simulink model "SmallFixedWingUAVupperHIL"  (R2022b)
settings: Solver=FixedStepDiscrete  StartTime=0.0  StopTime=inf  FixedStep=1/300  RelTol=1e-3
model workspace: external: MAT-File E:\RFLY\small-fixed-wing-book\fixedwing-book-rfly\ch8\code\e7-4\hitl\desire.mat (data not in the file)
values from neighbouring files (symbols this model uses):
  ctrlpoints = [xd'-xd(1);yd'-yd(1)]    [bspline.m]
  env = struct    [InitDatactrl.m]
  knots = [t1, t2, t3]    [bspline.m]
  pp = 3    [bspline.m]
  uav = struct    [InitDatactrl.m]
undefined symbols (not defined in the file or in its folder): DiscIntNeverNeededParam, RGBLED_COLOR_ENUM, RGBLED_MODE_ENUM
libraries: simulink x10, pixhawk_slib_sensors_actuators x6, pixhawk_slib_uORB_RW x5
(part 1 of 2)
settings Model: Creator=Steve  LastModifiedBy=DELL
settings SolverCC: AlgebraicLoopSolver=TrustRegion  AutoInsertRateTranBlk=on
settings DataIOCC: LimitDataPoints=on  SaveFormat=Array  ReturnWorkspaceOutputs=off
settings OptimizationCC: DefaultParameterBehavior=Inlined  ZeroExternalMemoryAtStartup=off  ZeroInternalMemoryAtStartup=off  LifeSpan=1  MaxStackSize=64  EfficientTunableParamExpr=on
settings DebuggingCC: SolverPrmCheckMsg=warning  UnconnectedInputMsg=warning  UnconnectedOutputMsg=warning  UnconnectedLineMsg=warning  AllowSymbolicDim=off  SFUnexpectedBacktrackingDiag=warning  SFNoUnconditionalDefaultTransitionDiag=warning  SFExecutionAtInitializationDiag=none  SFMachineParentedDataDiag=warning  ArithmeticOperatorsInVariantConditions=warning
settings HardwareCC: ProdBitPerPointer=32  ProdBitPerSizeT=32  ProdBitPerPtrDiffT=32  ProdLargestAtomicInteger=Long  ProdLargestAtomicFloat=Double  ProdWordSize=32  ProdHWDeviceType=ARM Compatible->ARM Cortex
settings ModelReferenceCC: EnableRefExpFcnMdlSchedulingChecks=on  PropagateSignalLabelsOutOfModel=off
settings SFSimCC: SimUseLocalCustomCode=off  MATLABDynamicMemAllocThreshold=0  CustomCodeUndefinedFunction=UseInterfaceOnly
settings RTWCC: Description=Embedded Coder  SystemTargetFile=ert.tlc  HardwareBoard=Pixhawk PX4  TemplateMakefile=ert_default_tmf  GenerateReport=on  RTWUseLocalCustomCode=off  Toolchain=Pixhawk Toolchain  BuildConfiguration=Faster Runs  IncludeHyperlinkInReport=on  LaunchReport=on  GenerateTraceReport=on  GenerateTraceReportSl=on  GenerateTraceReportSf=on  GenerateTraceReportEml=on  GenerateCodeMetricsReport=on  DLArmComputeVersion=19.05
settings CodeAppCC: IgnoreCustomStorageClasses=off  StateflowObjectComments=on
settings ERTTargetCC: TargetLangStandard=C99 (ISO)  CodeReplacementLibrary=GCC ARM Cortex-A9  MultiwordLength=2048  SupportContinuousTime=on  SupportVariableSizeSignals=on  ExtModeTransport=1  ExtModeMexFile=ext_serial_win32_comm  ExtModeMexArgs=/dev/serial  RootIOFormat=Structure reference  ERTCustomFileTemplate=PX4_codertarget_file_process.tlc  ConvertIfToSwitch=off  SuppressUnreachableDefaultCases=off
settings ConfigComp: CovMetricSettings=dw  CovSaveCumulativeToWorkspaceVar=on  CovSaveSingleToWorkspaceVar=on  CovExternalEMLEnable=off  CovSFcnEnable=off

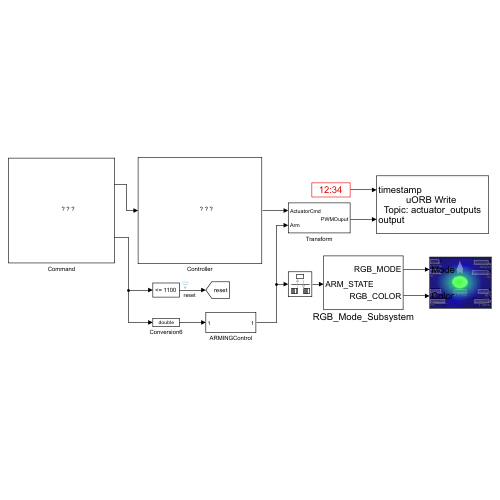
[thumbnail: Simulink's stored preview of the top-level diagram]
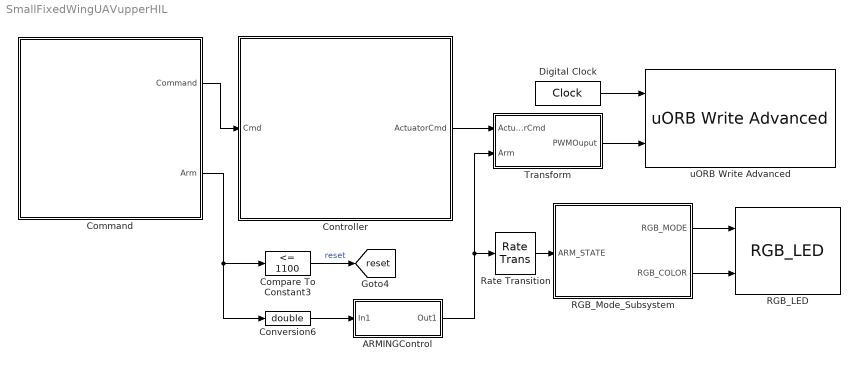
== system SmallFixedWingUAVupperHIL ==
  ARMINGControl : Subsystem
  Command : Subsystem
      mask Display: image('D:\GwhBuaa207\Project\2022-2023FW\fixedwing-book-rfly\chr\code\e0\hil\control\icon\ledi.jpg'); % 使用工具条上的 "编辑图像" 进行更改。
  Compare To Constant3 : simulink/Logic and Bit Operations/Compare To Constant  relop=<=  const=1100  OutDataTypeStr=boolean
  Controller : Subsystem
      mask Display: image('D:\GwhBuaa207\Project\2022-2023FW\fixedwing-book-rfly\chr\code\e0\hil\control\icon\Cube-Orange.jpg'); % 使用工具条上的 "编辑图像" 进行更改。
  Conversion6 : DataTypeConversion  OutDataTypeStr=double  SaturateOnIntegerOverflow=off  RndMeth=Floor
  Digital Clock : DigitalClock  SampleTime=-1
  RGB_LED : pixhawk_slib_sensors_actuators/RGB_LED
      settings: SourceProductName=Pixhawk Target Blocks
  RGB_Mode_Subsystem : Subsystem
  Rate Transition : RateTransition  OutPortSampleTime=1
  Transform : Subsystem
  uORB Write Advanced : pixhawk_slib_uORB_RW/uORB Write Advanced  Ts=0  uORB_AdvtQueue=on  uORB_FieldEnabledArr="0  0  0  1  0  0  0  0  0  0  0"  uORB_Topic_str=0  uORB_Struct_DT="[1  1  1  1  1]"  BlockInputCount=5  uORB_StructParams="[\"voltage_v\",\"voltage_filtered_v\",\"current_a\",\"current_filtered_a\",\"remaining\"]"  uORB_PortSizes="[1  1  1  1]"  MsgSizeOf=0  MW_update=true
      settings: SourceProductName=Pixhawk Target Blocks
  tag scope: reset=global
  wires:
  Digital Clock/1 -> uORB Write Advanced/1
  RGB_Mode_Subsystem/1(RGB_MODE) -> RGB_LED/1
  Rate Transition/1 -> RGB_Mode_Subsystem/1(ARM_STATE)
  ARMINGControl/1(Out1) -> Transform/2(Arm), Rate Transition/1
  RGB_Mode_Subsystem/2(RGB_COLOR) -> RGB_LED/2
  Conversion6/1 -> ARMINGControl/1(In1)
  Compare To Constant3/1 -> [reset]  "reset"
  Transform/1(PWMOuput) -> uORB Write Advanced/2
  Controller/1(ActuatorCmd) -> Transform/1(ActuatorCmd)
  Command/2(Arm) -> Conversion6/1, Compare To Constant3/1
  Command/1(Command) -> Controller/1(Cmd)

== system SmallFixedWingUAVupperHIL/ARMINGControl ==
  In1 : Inport
  Compare To Constant3 : simulink/Logic and Bit Operations/Compare To Constant  relop=>=  const=uint16(1500)  OutDataTypeStr=boolean
  Out1 : Outport  VectorParamsAs1DForOutWhenUnconnected=off
  wires:
  Compare To Constant3/1 -> Out1/1
  In1/1 -> Compare To Constant3/1

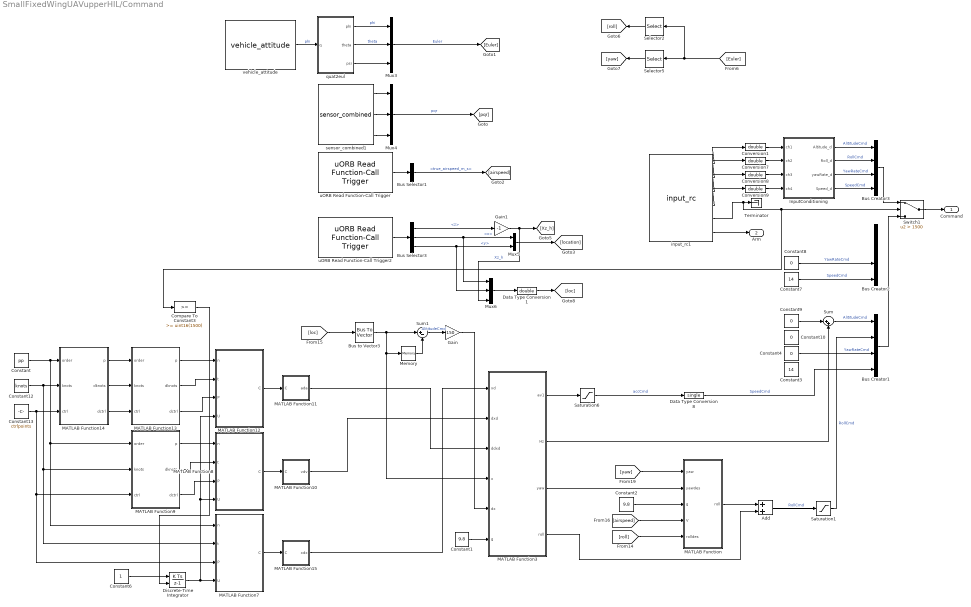
== system SmallFixedWingUAVupperHIL/Command ==
  Add : Sum
  Bus Creator1 : BusCreator  Inputs=4
  Bus Creator2 : BusCreator  Inputs=4
  Bus Creator3 : BusCreator  Inputs=4
  Bus Selector1 : BusSelector  OutputSignals=true_airspeed_m_s
  Bus Selector3 : BusSelector  OutputSignals=z,x,y
  Bus to Vector3 : BusToVector
  Compare To Constant3 : simulink/Logic and Bit Operations/Compare To Constant  relop=>=  const=uint16(1500)  OutDataTypeStr=boolean
  Constant : Constant  Value=pp
  Constant1 : Constant  Value=9.8
  Constant{4,8..10} (4 alike) : Constant  Value=0  SampleTime=-1
  Constant12 : Constant  Value=knots
  Constant13 : Constant  Value=ctrlpoints
  Constant2 : Constant  Value=9.8  SampleTime=-1
  Constant3 : Constant  Value=14  SampleTime=-1
  Constant6 : Constant
  Constant7 : Constant  Value=14  SampleTime=-1
  Conversion{1,7..9} (4 alike) : DataTypeConversion  OutDataTypeStr=double  SaturateOnIntegerOverflow=off  RndMeth=Floor
  Data Type Conversion1 : DataTypeConversion  OutDataTypeStr=double  SaturateOnIntegerOverflow=off  RndMeth=Floor
  Data Type Conversion8 : DataTypeConversion  OutDataTypeStr=single  SaturateOnIntegerOverflow=off  RndMeth=Floor
  Discrete-Time Integrator : DiscreteIntegrator  ExternalReset=either  SampleTime=-1  ICPrevOutput=DiscIntNeverNeededParam  ICPrevScaledInput=DiscIntNeverNeededParam
  Gain : Gain  Gain=150
  Gain1 : Gain  Gain=-1
  InputConditioning : Subsystem
  MATLAB Function : MATLAB Function  TreatAsAtomicUnit=on
  MATLAB Function10 : MATLAB Function  TreatAsAtomicUnit=on
  MATLAB Function11 : MATLAB Function  TreatAsAtomicUnit=on
  MATLAB Function12 : MATLAB Function  TreatAsAtomicUnit=on
  MATLAB Function13 : MATLAB Function  TreatAsAtomicUnit=on
  MATLAB Function14 : MATLAB Function  TreatAsAtomicUnit=on
  MATLAB Function15 : MATLAB Function  TreatAsAtomicUnit=on
  MATLAB Function3 : MATLAB Function  TreatAsAtomicUnit=on
  MATLAB Function7 : MATLAB Function  TreatAsAtomicUnit=on
  MATLAB Function8 : MATLAB Function  TreatAsAtomicUnit=on
  MATLAB Function9 : MATLAB Function  TreatAsAtomicUnit=on
  Memory : Memory  InheritSampleTime=on
  Mux3 : Mux  Inputs=3
  Mux4 : Mux  Inputs=3
  Mux5 : Mux  Inputs=2
  Mux6 : Mux  Inputs=3
  Saturation1 : Saturate  UpperLimit=0.4  LowerLimit=-0.4
  Saturation6 : Saturate  UpperLimit=10  LowerLimit=-10
  Selector2 : Selector  InputPortWidth=3  IndexOptions=Index vector (dialog)  Indices=1  OutputSizes=1
  Selector5 : Selector  InputPortWidth=3  IndexOptions=Index vector (dialog)  Indices=3  OutputSizes=1
  Sum : Sum  Inputs=|++
  Sum1 : Sum  Inputs=|+-
  Switch1 : Switch  Criteria=u2 > Threshold  Threshold=1500  SaturateOnIntegerOverflow=off  InputSameDT=off
  Terminator : Terminator
  input_rc1 : pixhawk_slib_sensors_actuators/input_rc  Description=|  sampletime=1/300  channel1=on  channel2=on  channel3=on  channel4=on  channel5=on  channel6=on  channel7=off  channel8=off  channel9=off  channel10=off  channel11=off  channel12=off  channel13=off  channel14=off  channel15=off  channel16=off  channel17=off  channel18=off  ch_count=off  rssi=off  rc_failsafe=off  rc_lost=off  rc_inputsource=off
      | RC Input Block
      | 
      | This block provides user input control to the model.
      | It uses the input_rc uORB topic.
      | 
      | The user has the ability to choose which channels are available as outputs from this block and also some optional outputs. These include 
      | Channels 1 through 18
      | double data type indicating the PWM value from the controller 
      | measured pulse widths for each of the supported channels 
      | Channel Count 
      | uint32 data type of the number of channels which are detector by the PX4 
      | RC Failsafe 
      | boolean data types indicating that the RC Tx is sending the FailSafe signal (if equipped and properly setup) 
      | explicit failsafe flag: true on TX failure or TX out of range , false otherwise. 
      | Only the true state is reliable, as there are some (PPM) receivers on the market going into failsafe without telling us explicitly. 
      | RC Input Source 
      | Enumeration data type indicating which source the RC input is from. 
      | Valid values are found in the ENUM file: RC_INPUT_SOURCE_ENUM.m 
      |           Enumeration members for class 'RC_INPUT_SOURCE_ENUM':
      |           RCINPUT_SOURCE_UNKNOWN         (0)
      |           RCINPUT_SOURCE_PX4FMU_PPM      (1)
      |           RCINPUT_SOURCE_PX4IO_PPM       (2)
      |           RCINPUT_SOURCE_PX4IO_SPEKTRUM  (3)
      |           RCINPUT_SOURCE_PX4IO_SBUS      (4)
      |           RCINPUT_SOURCE_PX4IO_ST24      (5)
      |           RCINPUT_SOURCE_MAVLINK         (6)
      |           RCINPUT_SOURCE_QURT            (7)
      |           RCINPUT_SOURCE_PX4FMU_SPEKTRUM (8)
      |           RCINPUT_SOURCE_PX4FMU_SBUS     (9)
      |           RCINPUT_SOURCE_PX4FMU_ST24     (10)
      |           RCINPUT_SOURCE_PX4FMU_SUMD     (11)
      |           RCINPUT_SOURCE_PX4FMU_DSM      (12)
      |           RCINPUT_SOURCE_PX4IO_SUMD      (13)
      | 
      | RSSI - Receive signal strength index 
      | receive signal strength indicator (RSSI): < 0: Undefined, 0: no signal, 255: full reception 
      | RC Lost Connection 
      | boolean data type indicating RC receiver connection status 
      | True, if no frame has arrived in the expected time, false otherwise. 
      | True usally means that the receiver has been disconnected, but can also indicate a radio link loss on "stupid" systems. 
      | Will remain false, if a RX with failsafe option continues to transmit frames after a link loss. 
      |   
      | Sample Model: px4demo_input_rc.slx
      settings: SourceProductName=Pixhawk Target Blocks
  quat2eul : MATLAB Function  TreatAsAtomicUnit=on
  sensor_combined1 : pixhawk_slib_sensors_actuators/sensor_combined  Description=|  sampletime=1/300  show_mag=off  show_acc=off  show_gyro=on  show_baro=off  show_ts=off
      | Sensor Combined Block
      | 
      | This block enables access to the various sensors available on the px4fmu-v2 hardware.  
      | The user can use these signals in the Simulink control model.  
      | The sample time needs to be provided in the mask dialog.  
      | Optional output ports can also be selected.  
      | Refer to the sample model: px4demo_attitude_control.slx
      | 
      | Signal definitions: 
      | Magnetometer (x,y,z) - single values – Magnetic field in NED body frame, in Gauss 
      | Accelerometer (x,y,z) - single values – Acceleration in NED body frame, in m/s^2 
      | Gyroscope (p,q,r) - single values – Angular velocity in radians per second 
      | Barometer (Altitude) - single value – Barometric pressure, already temperature compensated (millibars) 
      | RunTime (timestamp) - double value – Timestamp in microseconds since boot, from gyro 
      |   
      | The sensor_combined block needs to have the px4io service running on the PX4 hardware in order to get valid signal values.
      settings: SourceProductName=Pixhawk Target Blocks
  uORB Read Function-Call Trigger : pixhawk_slib_uORB_RW/uORB Read Function-Call Trigger  uORB_Topic_str='airspeed'  BusObjVar=Bus: airspeed_SL  uORB_Interval=1  AsyncOutput=off  Fcn_call_select=Generate Function Call Signal  TaskName='Task1'  Poll_timeout=100  Ts=-1
      settings: SourceProductName=Pixhawk Target Blocks
  uORB Read Function-Call Trigger2 : pixhawk_slib_uORB_RW/uORB Read Function-Call Trigger  uORB_Topic_str='vehicle_local_position'  BusObjVar=Bus: vehicle_local_position_SL  uORB_Interval=1  AsyncOutput=off  Fcn_call_select=Generate Function Call Signal  TaskName='Task1'  Poll_timeout=100  Ts=-1
      settings: SourceProductName=Pixhawk Target Blocks
  vehicle_attitude : pixhawk_slib_sensors_actuators/vehicle_attitude  sampletime=1/300  show_r=off  show_p=off  show_y=off  show_q=on  show_ts=off
      settings: SourceProductName=Pixhawk Target Blocks
  Command : Outport  VectorParamsAs1DForOutWhenUnconnected=off
  Arm : Outport  Port=2  VectorParamsAs1DForOutWhenUnconnected=off
  wires:
  InputConditioning/3(yawRate_d) -> Bus Creator3/3  "YawRateCmd"
  input_rc1/3 -> Conversion8/1
  input_rc1/2 -> Conversion7/1
  Conversion9/1 -> InputConditioning/4(ch4)
  InputConditioning/2(Roll_d) -> Bus Creator3/2  "RollCmd"
  Constant8/1 -> Bus Creator2/3  "YawRateCmd"
  input_rc1/4 -> Conversion9/1
  InputConditioning/4(Speed_d) -> Bus Creator3/4  "SpeedCmd"
  Conversion1/1 -> InputConditioning/1("ch1 ")
  InputConditioning/1(Altitude_d) -> Bus Creator3/1  "AlititudeCmd"
  input_rc1/5 -> Compare To Constant3/1, Switch1/2, Terminator/1
  Conversion8/1 -> InputConditioning/3(ch3)
  Constant7/1 -> Bus Creator2/4  "SpeedCmd"
  Bus Creator3/1 -> Switch1/1
  input_rc1/1 -> Conversion1/1
  Conversion7/1 -> InputConditioning/2(ch2)
  Switch1/1 -> Command/1
  input_rc1/6 -> Arm/1
  MATLAB Function3/4(roll) -> Add/2
  Saturation6/1 -> Data Type Conversion8/1  "accCmd"
  [airspeed] -> MATLAB Function/4(V)
  MATLAB Function3/3(yaw) -> MATLAB Function/2(yawdes)
  Bus to Vector3/1 -> Sum1/1, Memory/1, MATLAB Function3/4(x)
  Constant2/1 -> MATLAB Function/3(g)
  Constant1/1 -> MATLAB Function3/6(g)
  MATLAB Function/1(roll) -> Add/1
  MATLAB Function3/1(av1) -> Saturation6/1
  [loc] -> Bus to Vector3/1
  [roll] -> MATLAB Function/5(rolldes)
  [yaw] -> MATLAB Function/1(yaw)
  sensor_combined1/3 -> Mux4/3
  Mux4/1 -> [pqr]  "pqr"
  Mux3/1 -> [Euler]  "Euler"
  quat2eul/1(phi) -> Mux3/1  "phi"
  uORB Read Function-Call Trigger/1 -> Bus Selector1/1
  Bus Selector1/1 -> [airspeed]  "<true_airspeed_m_s>"
  vehicle_attitude/1 -> quat2eul/1(q)  "phi"
  quat2eul/2(theta) -> Mux3/2  "theta"
  sensor_combined1/2 -> Mux4/2
  sensor_combined1/1 -> Mux4/1
  quat2eul/3(psi) -> Mux3/3
  Mux6/1 -> Data Type Conversion1/1
  Bus Selector3/2 -> Mux6/1, Mux5/1  "<x>"
  Bus Selector3/3 -> Mux6/2, Mux5/2  "<y>"
  Bus Selector3/1 -> Gain1/1  "<z>"
  Gain1/1 -> Mux6/3, [Xz_h]  "Xz_h"
  Mux5/1 -> [location]
  uORB Read Function-Call Trigger2/1 -> Bus Selector3/1
  Data Type Conversion1/1 -> [loc]
  Selector2/1 -> [roll]
  Selector5/1 -> [yaw]
  [Euler] -> Selector2/1, Selector5/1
  Add/1 -> Saturation1/1  "RollCmd"
  Sum/1 -> Bus Creator1/1  "AlititudeCmd"
  Constant4/1 -> Bus Creator1/3  "YawRateCmd"
  Constant9/1 -> Sum/1
  Data Type Conversion8/1 -> Bus Creator1/4  "SpeedCmd"
  Bus Creator1/1 -> Switch1/3
  Memory/1 -> Sum1/2
  Sum1/1 -> Gain/1  "AlititudeCmd"
  Gain/1 -> MATLAB Function3/5(dx)
  MATLAB Function3/2(Hz) -> Sum/2
  Constant6/1 -> Discrete-Time Integrator/1
  Saturation1/1 -> Bus Creator1/2  "RollCmd"
  MATLAB Function8/1(C) -> MATLAB Function10/1(C)
  MATLAB Function7/1(C) -> MATLAB Function15/1(C)
  Constant13/1 -> MATLAB Function9/3(ctrl), MATLAB Function7/3(P), MATLAB Function14/3(ctrl)
  MATLAB Function14/2(dknots) -> MATLAB Function13/2(knots)
  MATLAB Function9/1(p) -> MATLAB Function8/1(n)
  MATLAB Function9/2(dknots) -> MATLAB Function8/2(t)
  MATLAB Function14/1(p) -> MATLAB Function13/1(order)
  Discrete-Time Integrator/1 -> MATLAB Function12/4(U), MATLAB Function8/4(U), MATLAB Function7/4(U)
  MATLAB Function12/1(C) -> MATLAB Function11/1(C)
  MATLAB Function14/3(dctrl) -> MATLAB Function13/3(ctrl)
  MATLAB Function13/3(dctrl) -> MATLAB Function12/3(P)
  Constant12/1 -> MATLAB Function9/2(knots), MATLAB Function7/2(t), MATLAB Function14/2(knots)
  MATLAB Function13/1(p) -> MATLAB Function12/1(n)
  MATLAB Function13/2(dknots) -> MATLAB Function12/2(t)
  MATLAB Function9/3(dctrl) -> MATLAB Function8/3(P)
  Constant/1 -> MATLAB Function9/1(order), MATLAB Function7/1(n), MATLAB Function14/1(order)
  Compare To Constant3/1 -> Discrete-Time Integrator/2
  MATLAB Function11/1(ada) -> MATLAB Function3/3(ddxd)
  MATLAB Function10/1(vdv) -> MATLAB Function3/2(dxd)
  MATLAB Function15/1(xdx) -> MATLAB Function3/1(xd)

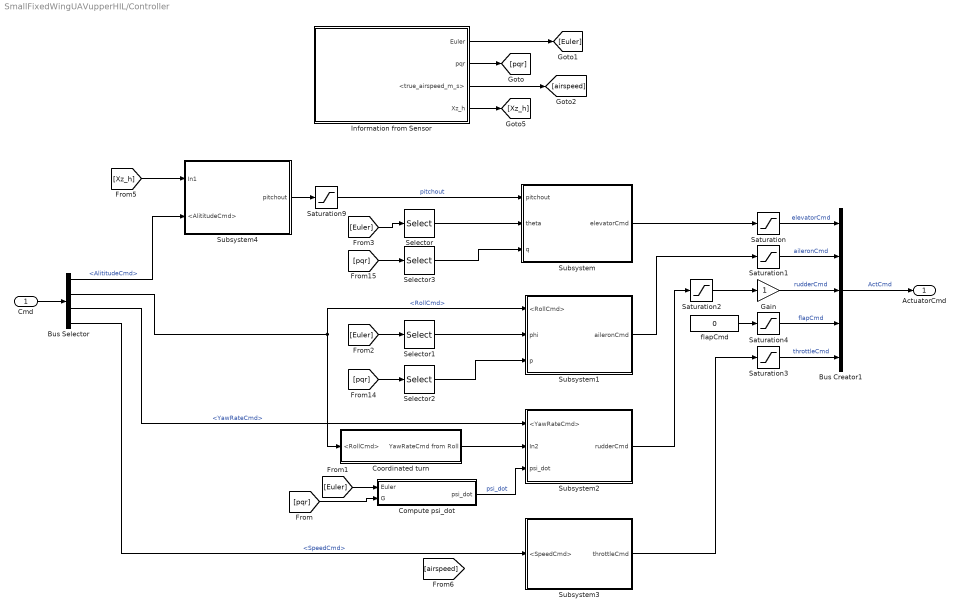
== system SmallFixedWingUAVupperHIL/Controller ==
  Cmd : Inport
  Bus Creator1 : BusCreator  Inputs=5
  Bus Selector : BusSelector  OutputSignals=AlititudeCmd,RollCmd,YawRateCmd,SpeedCmd
  Compute psi_dot : Subsystem
  Coordinated turn : Subsystem
  Gain : Gain
  Information from Sensor : Subsystem
  Saturation : Saturate  UpperLimit=uav.elevator.max  LowerLimit=uav.elevator.min
  Saturation1 : Saturate  UpperLimit=uav.aileron.max  LowerLimit=uav.aileron.min
  Saturation2 : Saturate  UpperLimit=uav.rudder.max  LowerLimit=uav.rudder.min
  Saturation3 : Saturate  UpperLimit=uav.throttlepercent.max  LowerLimit=uav.throttlepercent.min
  Saturation4 : Saturate  UpperLimit=uav.flap.max  LowerLimit=uav.flap.min
  Saturation9 : Saturate  UpperLimit=uav.attitudectrlmax.pitch  LowerLimit=-uav.attitudectrlmax.pitch
  Selector : Selector  InputPortWidth=3  IndexOptions=Index vector (dialog)  Indices=2  OutputSizes=1
  Selector1 : Selector  InputPortWidth=3  IndexOptions=Index vector (dialog)  Indices=1  OutputSizes=1
  Selector2 : Selector  InputPortWidth=3  IndexOptions=Index vector (dialog)  Indices=1  OutputSizes=1
  Selector3 : Selector  InputPortWidth=3  IndexOptions=Index vector (dialog)  Indices=2  OutputSizes=1
  Subsystem : Subsystem
  Subsystem1 : Subsystem
  Subsystem2 : Subsystem
  Subsystem3 : Subsystem
  Subsystem4 : Subsystem
  flapCmd : Constant  Value=0  OutDataTypeStr=double
  ActuatorCmd : Outport  VectorParamsAs1DForOutWhenUnconnected=off
  wires:
  [Euler] -> Selector/1
  Saturation9/1 -> Subsystem/1(pitchout)  "pitchout"
  Selector1/1 -> Subsystem1/2(phi)
  Bus Selector/4 -> Subsystem3/1(<SpeedCmd>)  "<SpeedCmd>"
  Bus Selector/3 -> Subsystem2/1(<YawRateCmd>)  "<YawRateCmd>"
  Bus Selector/1 -> Subsystem4/2(<AlititudeCmd>)  "<AlititudeCmd>"
  Saturation2/1 -> Gain/1
  [pqr] -> Selector2/1
  Subsystem1/1(aileronCmd) -> Saturation1/1
  Information from Sensor/1(Euler) -> [Euler]
  Subsystem2/1(rudderCmd) -> Saturation2/1
  Compute psi_dot/1(psi_dot) -> Subsystem2/3(psi_dot)  "psi_dot"
  Saturation3/1 -> Bus Creator1/5  "throttleCmd"
  Coordinated turn/1(YawRateCmd from Roll) -> Subsystem2/2(In2)
  Selector/1 -> Subsystem/2(theta)
  [Euler] -> Compute psi_dot/1(Euler)
  [Euler] -> Selector1/1
  Subsystem3/1(throttleCmd) -> Saturation3/1
  Bus Selector/2 -> Coordinated turn/1(<RollCmd>), Subsystem1/1(<RollCmd>)  "<RollCmd>"
  [Xz_h] -> Subsystem4/1(In1)
  Selector2/1 -> Subsystem1/3(p)
  Gain/1 -> Bus Creator1/3  "rudderCmd"
  Information from Sensor/3(<true_airspeed_m_s>) -> [airspeed]
  [pqr] -> Selector3/1
  Subsystem4/1(pitchout) -> Saturation9/1
  flapCmd/1 -> Saturation4/1
  [pqr] -> Compute psi_dot/2(G)
  Selector3/1 -> Subsystem/3(q)
  Cmd/1 -> Bus Selector/1
  Information from Sensor/2(pqr) -> [pqr]
  Information from Sensor/4(Xz_h) -> [Xz_h]
  Saturation/1 -> Bus Creator1/1  "elevatorCmd"
  Subsystem/1(elevatorCmd) -> Saturation/1
  Saturation4/1 -> Bus Creator1/4  "flapCmd"
  Saturation1/1 -> Bus Creator1/2  "aileronCmd"
  Bus Creator1/1 -> ActuatorCmd/1  "ActCmd"

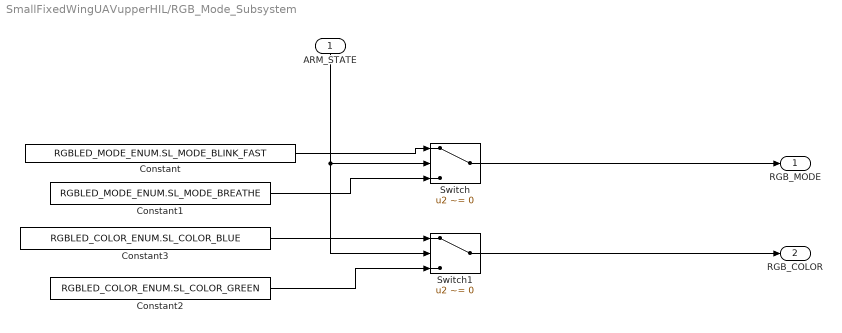
== system SmallFixedWingUAVupperHIL/RGB_Mode_Subsystem ==
  ARM_STATE : Inport
  Constant : Constant  Value=RGBLED_MODE_ENUM.SL_MODE_BLINK_FAST  OutDataTypeStr=Enum: RGBLED_MODE_ENUM
  Constant1 : Constant  Value=RGBLED_MODE_ENUM.SL_MODE_BREATHE  OutDataTypeStr=Enum: RGBLED_MODE_ENUM
  Constant2 : Constant  Value=RGBLED_COLOR_ENUM.SL_COLOR_GREEN  OutDataTypeStr=Enum: RGBLED_COLOR_ENUM
  Constant3 : Constant  Value=RGBLED_COLOR_ENUM.SL_COLOR_BLUE  OutDataTypeStr=Enum: RGBLED_COLOR_ENUM
  Switch : Switch  Criteria=u2 ~= 0  Threshold=1500  SaturateOnIntegerOverflow=off  InputSameDT=off
  Switch1 : Switch  Criteria=u2 ~= 0  Threshold=1500  SaturateOnIntegerOverflow=off  InputSameDT=off
  RGB_MODE : Outport  VectorParamsAs1DForOutWhenUnconnected=off
  RGB_COLOR : Outport  Port=2  VectorParamsAs1DForOutWhenUnconnected=off
  wires:
  ARM_STATE/1 -> Switch1/2, Switch/2
  Constant/1 -> Switch/1
  Constant1/1 -> Switch/3
  Switch/1 -> RGB_MODE/1
  Constant3/1 -> Switch1/1
  Constant2/1 -> Switch1/3
  Switch1/1 -> RGB_COLOR/1

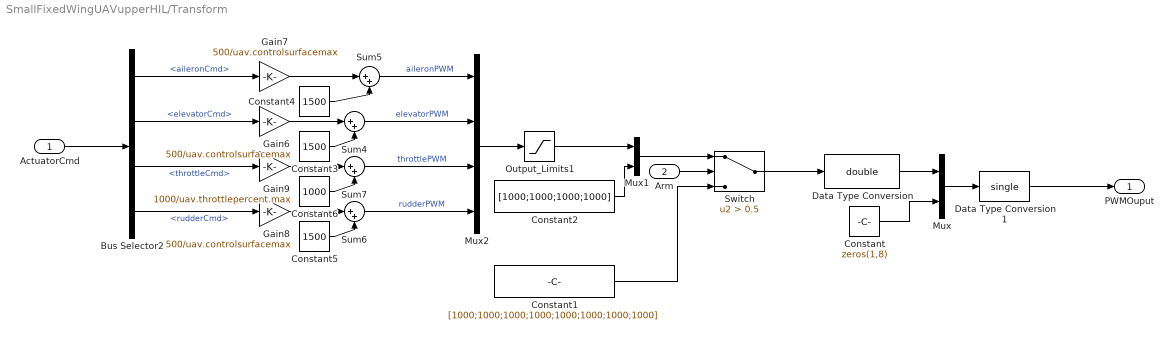
== system SmallFixedWingUAVupperHIL/Transform ==
  ActuatorCmd : Inport
  Arm : Inport  Port=2
  Bus Selector2 : BusSelector  OutputSignals=aileronCmd,elevatorCmd,throttleCmd,rudderCmd
  Constant : Constant  Value=zeros(1,8)
  Constant1 : Constant  Value=[1000;1000;1000;1000;1000;1000;1000;1000]
  Constant2 : Constant  Value=[1000;1000;1000;1000]
  Constant3 : Constant  Value=1500
  Constant4 : Constant  Value=1500
  Constant5 : Constant  Value=1500
  Constant6 : Constant  Value=1000
  Data Type Conversion : DataTypeConversion  OutDataTypeStr=double  SaturateOnIntegerOverflow=off  RndMeth=Floor
  Data Type Conversion1 : DataTypeConversion  OutDataTypeStr=single  SaturateOnIntegerOverflow=off  RndMeth=Floor
  Gain6 : Gain  Gain=500/uav.controlsurfacemax
  Gain7 : Gain  Gain=500/uav.controlsurfacemax
  Gain8 : Gain  Gain=500/uav.controlsurfacemax
  Gain9 : Gain  Gain=1000/uav.throttlepercent.max
  Mux : Mux  Inputs=2
  Mux1 : Mux  Inputs=2
  Mux2 : Mux
  Output_Limits1 : Saturate  UpperLimit=2000  LowerLimit=1000
  Sum{4..7} (4 alike) : Sum  Inputs=|++
  Switch : Switch  Criteria=u2 > Threshold  Threshold=0.5  SaturateOnIntegerOverflow=off  InputSameDT=off
  PWMOuput : Outport  VectorParamsAs1DForOutWhenUnconnected=off
  wires:
  Constant2/1 -> Mux1/2
  Sum6/1 -> Mux2/4  "rudderPWM"
  Data Type Conversion/1 -> Mux/1
  Bus Selector2/4 -> Gain8/1  "<rudderCmd>"
  Bus Selector2/2 -> Gain6/1  "<elevatorCmd>"
  Constant3/1 -> Sum4/2
  Switch/1 -> Data Type Conversion/1
  Gain6/1 -> Sum4/1
  Bus Selector2/3 -> Gain9/1  "<throttleCmd>"
  Bus Selector2/1 -> Gain7/1  "<aileronCmd>"
  Constant/1 -> Mux/2
  Gain8/1 -> Sum6/1
  Sum7/1 -> Mux2/3  "throttlePWM"
  Constant1/1 -> Switch/3
  Mux1/1 -> Switch/1
  Output_Limits1/1 -> Mux1/1
  Constant5/1 -> Sum6/2
  Sum5/1 -> Mux2/1  "aileronPWM"
  Sum4/1 -> Mux2/2  "elevatorPWM"
  Constant6/1 -> Sum7/2
  Mux2/1 -> Output_Limits1/1
  Gain7/1 -> Sum5/1
  Mux/1 -> Data Type Conversion1/1
  Gain9/1 -> Sum7/1
  Constant4/1 -> Sum5/2
  Arm/1 -> Switch/2
  ActuatorCmd/1 -> Bus Selector2/1
  Data Type Conversion1/1 -> PWMOuput/1

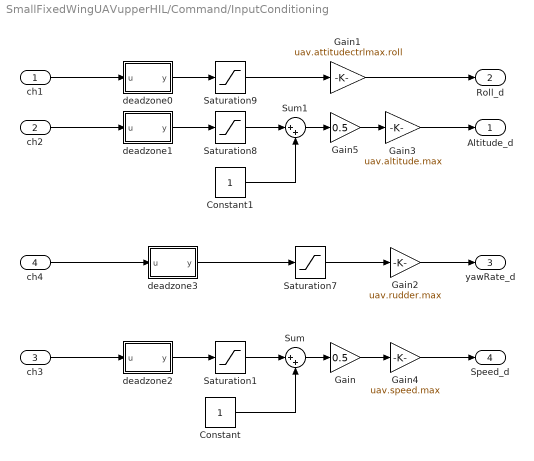
== system SmallFixedWingUAVupperHIL/Command/InputConditioning ==
  "ch1 " : Inport
  ch2 : Inport  Port=2
  ch3 : Inport  Port=3
  ch4 : Inport  Port=4
  Constant : Constant
  Constant1 : Constant
  Gain : Gain  Gain=0.5
  Gain1 : Gain  Gain=uav.attitudectrlmax.roll  OutDataTypeStr=Inherit: Inherit via back propagation
  Gain2 : Gain  Gain=uav.rudder.max
  Gain3 : Gain  Gain=uav.altitude.max  OutDataTypeStr=Inherit: Inherit via back propagation
  Gain4 : Gain  Gain=uav.speed.max
  Gain5 : Gain  Gain=0.5
  Saturation{1,7..9} (4 alike) : Saturate  UpperLimit=1  LowerLimit=-1
  Sum : Sum  Inputs=|++
  Sum1 : Sum  Inputs=|++
  deadzone0 : MATLAB Function  TreatAsAtomicUnit=on
  deadzone1 : MATLAB Function  TreatAsAtomicUnit=on
  deadzone2 : MATLAB Function  TreatAsAtomicUnit=on
  deadzone3 : MATLAB Function  TreatAsAtomicUnit=on
  Altitude_d : Outport  VectorParamsAs1DForOutWhenUnconnected=off
  Roll_d : Outport  Port=2  VectorParamsAs1DForOutWhenUnconnected=off
  yawRate_d : Outport  Port=3  VectorParamsAs1DForOutWhenUnconnected=off
  Speed_d : Outport  Port=4  VectorParamsAs1DForOutWhenUnconnected=off
  wires:
  deadzone2/1(y) -> Saturation1/1
  ch3/1 -> deadzone2/1(u)
  deadzone1/1(y) -> Saturation8/1
  Gain/1 -> Gain4/1
  deadzone0/1(y) -> Saturation9/1
  "ch1 "/1 -> deadzone0/1(u)
  ch2/1 -> deadzone1/1(u)
  Saturation9/1 -> Gain1/1
  Saturation8/1 -> Sum1/1
  Constant/1 -> Sum/2
  Sum/1 -> Gain/1
  Gain1/1 -> Roll_d/1
  Gain3/1 -> Altitude_d/1
  Saturation7/1 -> Gain2/1
  deadzone3/1(y) -> Saturation7/1
  ch4/1 -> deadzone3/1(u)
  Gain2/1 -> yawRate_d/1
  Saturation1/1 -> Sum/1
  Gain4/1 -> Speed_d/1
  Gain5/1 -> Gain3/1
  Constant1/1 -> Sum1/2
  Sum1/1 -> Gain5/1

== system SmallFixedWingUAVupperHIL/Controller/Compute psi_dot ==
  Euler : Inport
  G : Inport  Port=2
  Mux1 : Mux  Inputs=2
  psidot : Fcn  Expr=(u[5]*sin(u[1])+u[6]*cos(u[1]))/cos(u[2])
  psi_dot : Outport  Unit=rad/S  VectorParamsAs1DForOutWhenUnconnected=off
  wires:
  G/1 -> Mux1/2
  psidot/1 -> psi_dot/1  "psi_dot"
  Mux1/1 -> psidot/1
  Euler/1 -> Mux1/1

== system SmallFixedWingUAVupperHIL/Controller/Coordinated turn ==
  <RollCmd> : Inport
  Divide : Product  Inputs=*/*
  Trigonometric Function : Trigonometry  Operator=tan
  env.ISA_g : Constant  Value=env.ISA_g
  YawRateCmd from Roll : Outport  VectorParamsAs1DForOutWhenUnconnected=off
  wires:
  env.ISA_g/1 -> Divide/3
  [airspeed] -> Divide/2
  Trigonometric Function/1 -> Divide/1
  Divide/1 -> YawRateCmd from Roll/1  "YawRateCmd from Roll"
  <RollCmd>/1 -> Trigonometric Function/1

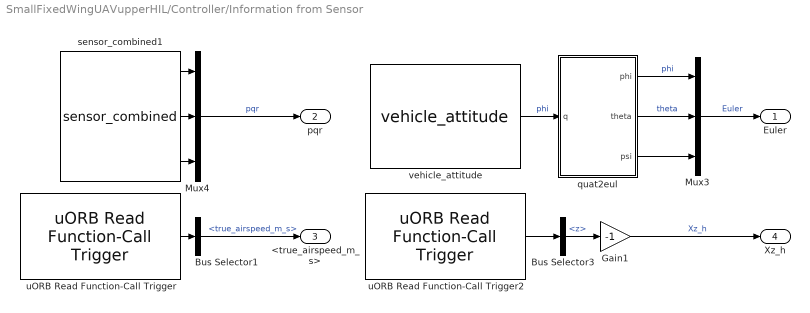
== system SmallFixedWingUAVupperHIL/Controller/Information from Sensor ==
  Bus Selector1 : BusSelector  OutputSignals=true_airspeed_m_s
  Bus Selector3 : BusSelector  OutputSignals=z
  Gain1 : Gain  Gain=-1
  Mux3 : Mux  Inputs=3
  Mux4 : Mux  Inputs=3
  quat2eul : MATLAB Function  TreatAsAtomicUnit=on
  sensor_combined1 : pixhawk_slib_sensors_actuators/sensor_combined  Description=|  sampletime=1/300  show_mag=off  show_acc=off  show_gyro=on  show_baro=off  show_ts=off
      | Sensor Combined Block
      | 
      | This block enables access to the various sensors available on the px4fmu-v2 hardware.  
      | The user can use these signals in the Simulink control model.  
      | The sample time needs to be provided in the mask dialog.  
      | Optional output ports can also be selected.  
      | Refer to the sample model: px4demo_attitude_control.slx
      | 
      | Signal definitions: 
      | Magnetometer (x,y,z) - single values – Magnetic field in NED body frame, in Gauss 
      | Accelerometer (x,y,z) - single values – Acceleration in NED body frame, in m/s^2 
      | Gyroscope (p,q,r) - single values – Angular velocity in radians per second 
      | Barometer (Altitude) - single value – Barometric pressure, already temperature compensated (millibars) 
      | RunTime (timestamp) - double value – Timestamp in microseconds since boot, from gyro 
      |   
      | The sensor_combined block needs to have the px4io service running on the PX4 hardware in order to get valid signal values.
      settings: SourceProductName=Pixhawk Target Blocks
  uORB Read Function-Call Trigger : pixhawk_slib_uORB_RW/uORB Read Function-Call Trigger  uORB_Topic_str='airspeed'  BusObjVar=Bus: airspeed_SL  uORB_Interval=1  AsyncOutput=off  Fcn_call_select=Generate Function Call Signal  TaskName='Task1'  Poll_timeout=100  Ts=-1
      settings: SourceProductName=Pixhawk Target Blocks
  uORB Read Function-Call Trigger2 : pixhawk_slib_uORB_RW/uORB Read Function-Call Trigger  uORB_Topic_str='vehicle_local_position'  BusObjVar=Bus: vehicle_local_position_SL  uORB_Interval=1  AsyncOutput=off  Fcn_call_select=Generate Function Call Signal  TaskName='Task1'  Poll_timeout=100  Ts=-1
      settings: SourceProductName=Pixhawk Target Blocks
  vehicle_attitude : pixhawk_slib_sensors_actuators/vehicle_attitude  sampletime=1/300  show_r=off  show_p=off  show_y=off  show_q=on  show_ts=off
      settings: SourceProductName=Pixhawk Target Blocks
  Euler : Outport  VectorParamsAs1DForOutWhenUnconnected=off
  pqr : Outport  Port=2  VectorParamsAs1DForOutWhenUnconnected=off
  <true_airspeed_m_s> : Outport  Port=3  VectorParamsAs1DForOutWhenUnconnected=off
  Xz_h : Outport  Port=4  VectorParamsAs1DForOutWhenUnconnected=off
  wires:
  sensor_combined1/2 -> Mux4/2
  Mux4/1 -> pqr/1  "pqr"
  Mux3/1 -> Euler/1  "Euler"
  Gain1/1 -> Xz_h/1  "Xz_h"
  Bus Selector1/1 -> <true_airspeed_m_s>/1  "<true_airspeed_m_s>"
  quat2eul/3(psi) -> Mux3/3
  quat2eul/1(phi) -> Mux3/1  "phi"
  vehicle_attitude/1 -> quat2eul/1(q)  "phi"
  uORB Read Function-Call Trigger/1 -> Bus Selector1/1
  uORB Read Function-Call Trigger2/1 -> Bus Selector3/1
  sensor_combined1/3 -> Mux4/3
  sensor_combined1/1 -> Mux4/1
  Bus Selector3/1 -> Gain1/1  "<z>"
  quat2eul/2(theta) -> Mux3/2  "theta"

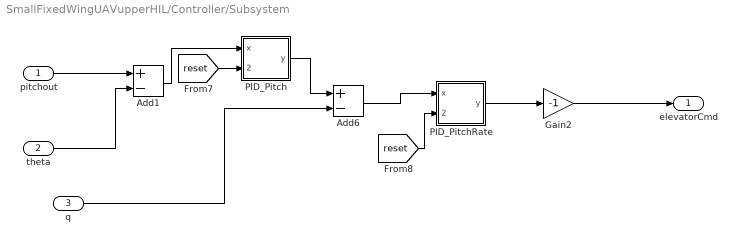
== system SmallFixedWingUAVupperHIL/Controller/Subsystem ==
  pitchout : Inport
  theta : Inport  Port=2
  q : Inport  Port=3
  Add1 : Sum  Inputs=+-
  Add6 : Sum  Inputs=+-
  Gain2 : Gain  Gain=-1
  PID_Pitch : Subsystem
  PID_PitchRate : Subsystem
  elevatorCmd : Outport  VectorParamsAs1DForOutWhenUnconnected=off
  wires:
  PID_PitchRate/1(y) -> Gain2/1
  q/1 -> Add6/2
  Add1/1 -> PID_Pitch/1(x)
  [reset] -> PID_PitchRate/2(reset_i)
  [reset] -> PID_Pitch/2(reset_i)
  theta/1 -> Add1/2
  PID_Pitch/1(y) -> Add6/1
  Add6/1 -> PID_PitchRate/1(x)
  Gain2/1 -> elevatorCmd/1
  pitchout/1 -> Add1/1

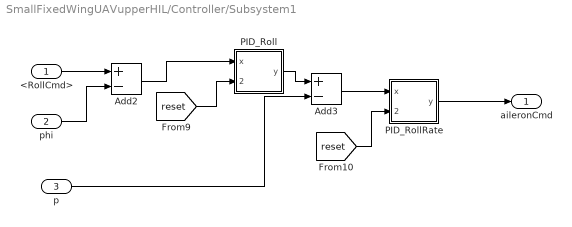
== system SmallFixedWingUAVupperHIL/Controller/Subsystem1 ==
  <RollCmd> : Inport
  phi : Inport  Port=2
  p : Inport  Port=3
  Add2 : Sum  Inputs=+-
  Add3 : Sum  Inputs=+-
  PID_Roll : Subsystem
  PID_RollRate : Subsystem
  aileronCmd : Outport  VectorParamsAs1DForOutWhenUnconnected=off
  wires:
  Add3/1 -> PID_RollRate/1(x)
  [reset] -> PID_Roll/2(reset_i)
  PID_Roll/1(y) -> Add3/1
  Add2/1 -> PID_Roll/1(x)
  [reset] -> PID_RollRate/2(reset_i)
  PID_RollRate/1(y) -> aileronCmd/1
  phi/1 -> Add2/2
  p/1 -> Add3/2
  <RollCmd>/1 -> Add2/1

== system SmallFixedWingUAVupperHIL/Controller/Subsystem2 ==
  <YawRateCmd> : Inport
  In2 : Inport  Port=2
  psi_dot : Inport  Port=3
  Add4 : Sum  Inputs=+-
  PID_YawRate : Subsystem
  Sum2 : Sum  Inputs=++|
  rudderCmd : Outport  VectorParamsAs1DForOutWhenUnconnected=off
  wires:
  Add4/1 -> PID_YawRate/1(x)
  [reset] -> PID_YawRate/2(reset_i)
  psi_dot/1 -> Add4/2
  PID_YawRate/1(y) -> Sum2/2
  <YawRateCmd>/1 -> Sum2/1
  Sum2/1 -> rudderCmd/1
  In2/1 -> Add4/1

== system SmallFixedWingUAVupperHIL/Controller/Subsystem3 ==
  <SpeedCmd> : Inport
  Add7 : Sum  Inputs=+-
  PID_Speed : Subsystem
  throttleCmd : Outport  VectorParamsAs1DForOutWhenUnconnected=off
  wires:
  [reset] -> PID_Speed/2(reset_i)
  Add7/1 -> PID_Speed/1(x)  "speederror"
  <SpeedCmd>/1 -> throttleCmd/1

== system SmallFixedWingUAVupperHIL/Controller/Subsystem4 ==
  In1 : Inport
  <AlititudeCmd> : Inport  Port=2
  Add8 : Sum  Inputs=+-
  PID_Altitude : Subsystem
  pitchout : Outport  VectorParamsAs1DForOutWhenUnconnected=off
  wires:
  [reset] -> PID_Altitude/2(reset_i)
  In1/1 -> Add8/2
  Add8/1 -> PID_Altitude/1(x)
  <AlititudeCmd>/1 -> Add8/1
  PID_Altitude/1(y) -> pitchout/1  "pitchout"

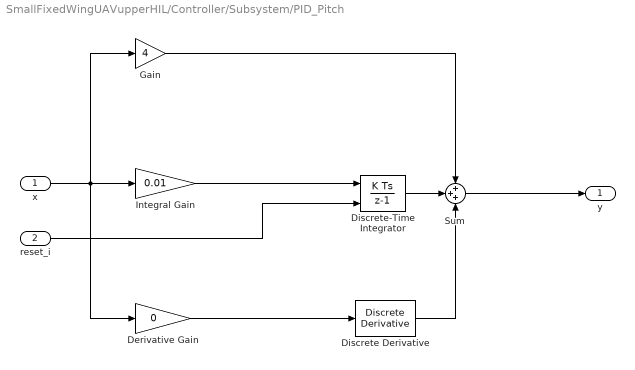
== system SmallFixedWingUAVupperHIL/Controller/Subsystem/PID_Pitch ==
  x : Inport
  reset_i : Inport  Port=2
  Derivative Gain : Gain  DisableCoverage=on  Gain=0  ParamMin=-100  ParamMax=100  OutMin=-100  OutMax=100
  Discrete Derivative : simulink/Discrete/Discrete Derivative  gainval=1.0  ICPrevScaledInput=0.0  OutMin=[]  OutMax=[]  OutDataType=fixdt(1, 16)  OutScaling=2^-10  DoSatur=off
  Discrete-Time Integrator : DiscreteIntegrator  ExternalReset=either  SampleTime=-1  ICPrevOutput=DiscIntNeverNeededParam  ICPrevScaledInput=DiscIntNeverNeededParam
  Gain : Gain  Gain=4
  Integral Gain : Gain  DisableCoverage=on  Gain=0.01
  Sum : Sum  Inputs=+++
  y : Outport  InitialOutput=0  VectorParamsAs1DForOutWhenUnconnected=off
  wires:
  reset_i/1 -> Discrete-Time Integrator/2
  Discrete-Time Integrator/1 -> Sum/2
  Discrete Derivative/1 -> Sum/3
  Sum/1 -> y/1
  Gain/1 -> Sum/1
  Derivative Gain/1 -> Discrete Derivative/1
  Integral Gain/1 -> Discrete-Time Integrator/1
  x/1 -> Derivative Gain/1, Integral Gain/1, Gain/1

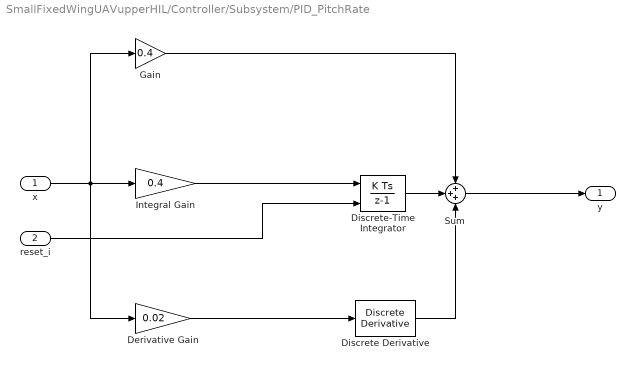
== system SmallFixedWingUAVupperHIL/Controller/Subsystem/PID_PitchRate ==
  x : Inport
  reset_i : Inport  Port=2
  Derivative Gain : Gain  DisableCoverage=on  Gain=0.02  ParamMin=-100  ParamMax=100  OutMin=-100  OutMax=100
  Discrete Derivative : simulink/Discrete/Discrete Derivative  gainval=1.0  ICPrevScaledInput=0.0  OutMin=[]  OutMax=[]  OutDataType=fixdt(1, 16)  OutScaling=2^-10  DoSatur=off
  Discrete-Time Integrator : DiscreteIntegrator  ExternalReset=either  SampleTime=-1  LimitOutput=on  UpperSaturationLimit=0.3  LowerSaturationLimit=-0.3  ICPrevOutput=DiscIntNeverNeededParam  ICPrevScaledInput=DiscIntNeverNeededParam
  Gain : Gain  Gain=0.4
  Integral Gain : Gain  DisableCoverage=on  Gain=0.4
  Sum : Sum  Inputs=+++
  y : Outport  InitialOutput=0  VectorParamsAs1DForOutWhenUnconnected=off
  wires:
  x/1 -> Gain/1, Integral Gain/1, Derivative Gain/1
  Integral Gain/1 -> Discrete-Time Integrator/1
  Derivative Gain/1 -> Discrete Derivative/1
  Gain/1 -> Sum/1
  Sum/1 -> y/1
  Discrete Derivative/1 -> Sum/3
  Discrete-Time Integrator/1 -> Sum/2
  reset_i/1 -> Discrete-Time Integrator/2

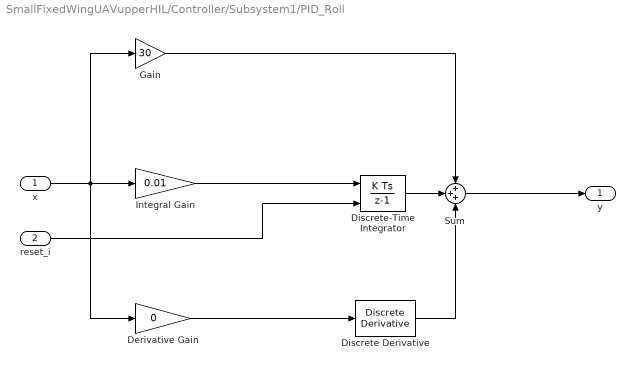
== system SmallFixedWingUAVupperHIL/Controller/Subsystem1/PID_Roll ==
  x : Inport
  reset_i : Inport  Port=2
  Derivative Gain : Gain  DisableCoverage=on  Gain=0  ParamMin=-100  ParamMax=100  OutMin=-100  OutMax=100
  Discrete Derivative : simulink/Discrete/Discrete Derivative  gainval=1.0  ICPrevScaledInput=0.0  OutMin=[]  OutMax=[]  OutDataType=fixdt(1, 16)  OutScaling=2^-10  DoSatur=off
  Discrete-Time Integrator : DiscreteIntegrator  ExternalReset=either  SampleTime=-1  ICPrevOutput=DiscIntNeverNeededParam  ICPrevScaledInput=DiscIntNeverNeededParam
  Gain : Gain  Gain=30
  Integral Gain : Gain  DisableCoverage=on  Gain=0.01
  Sum : Sum  Inputs=+++
  y : Outport  InitialOutput=0  VectorParamsAs1DForOutWhenUnconnected=off
  wires:
  x/1 -> Gain/1, Integral Gain/1, Derivative Gain/1
  Integral Gain/1 -> Discrete-Time Integrator/1
  Derivative Gain/1 -> Discrete Derivative/1
  Gain/1 -> Sum/1
  Sum/1 -> y/1
  Discrete Derivative/1 -> Sum/3
  Discrete-Time Integrator/1 -> Sum/2
  reset_i/1 -> Discrete-Time Integrator/2

== system SmallFixedWingUAVupperHIL/Controller/Subsystem1/PID_RollRate ==
  x : Inport
  reset_i : Inport  Port=2
  Derivative Gain : Gain  DisableCoverage=on  Gain=0.05  ParamMin=-100  ParamMax=100  OutMin=-100  OutMax=100
  Discrete Derivative : simulink/Discrete/Discrete Derivative  gainval=1.0  ICPrevScaledInput=0.0  OutMin=[]  OutMax=[]  OutDataType=fixdt(1, 16)  OutScaling=2^-10  DoSatur=off
  Discrete-Time Integrator : DiscreteIntegrator  ExternalReset=either  SampleTime=-1  LimitOutput=on  UpperSaturationLimit=0.3  LowerSaturationLimit=-0.3  ICPrevOutput=DiscIntNeverNeededParam  ICPrevScaledInput=DiscIntNeverNeededParam
  Gain : Gain
  Integral Gain : Gain  DisableCoverage=on  Gain=0.6
  Sum : Sum  Inputs=+++
  y : Outport  InitialOutput=0  VectorParamsAs1DForOutWhenUnconnected=off
  wires:
  reset_i/1 -> Discrete-Time Integrator/2
  Discrete-Time Integrator/1 -> Sum/2
  Discrete Derivative/1 -> Sum/3
  Sum/1 -> y/1
  Gain/1 -> Sum/1
  Derivative Gain/1 -> Discrete Derivative/1
  Integral Gain/1 -> Discrete-Time Integrator/1
  x/1 -> Derivative Gain/1, Integral Gain/1, Gain/1

== system SmallFixedWingUAVupperHIL/Controller/Subsystem2/PID_YawRate ==
  x : Inport
  reset_i : Inport  Port=2
  Derivative Gain : Gain  DisableCoverage=on  Gain=0.01  ParamMin=-100  ParamMax=100  OutMin=-100  OutMax=100
  Discrete Derivative : simulink/Discrete/Discrete Derivative  gainval=1.0  ICPrevScaledInput=0.0  OutMin=[]  OutMax=[]  OutDataType=fixdt(1, 16)  OutScaling=2^-10  DoSatur=off
  Discrete-Time Integrator : DiscreteIntegrator  ExternalReset=either  SampleTime=-1  LimitOutput=on  UpperSaturationLimit=0.3  LowerSaturationLimit=-0.3  ICPrevOutput=DiscIntNeverNeededParam  ICPrevScaledInput=DiscIntNeverNeededParam
  Gain : Gain  Gain=1.2
  Integral Gain : Gain  DisableCoverage=on  Gain=0.2
  Sum : Sum  Inputs=+++
  y : Outport  InitialOutput=0  VectorParamsAs1DForOutWhenUnconnected=off
  wires:
  x/1 -> Gain/1, Integral Gain/1, Derivative Gain/1
  Integral Gain/1 -> Discrete-Time Integrator/1
  Derivative Gain/1 -> Discrete Derivative/1
  Gain/1 -> Sum/1
  Sum/1 -> y/1
  Discrete Derivative/1 -> Sum/3
  Discrete-Time Integrator/1 -> Sum/2
  reset_i/1 -> Discrete-Time Integrator/2

== system SmallFixedWingUAVupperHIL/Controller/Subsystem3/PID_Speed ==
  x : Inport
  reset_i : Inport  Port=2
  Derivative Gain : Gain  DisableCoverage=on  Gain=0  ParamMin=-100  ParamMax=100  OutMin=-100  OutMax=100
  Discrete Derivative : simulink/Discrete/Discrete Derivative  gainval=1.0  ICPrevScaledInput=0.0  OutMin=[]  OutMax=[]  OutDataType=fixdt(1, 16)  OutScaling=2^-10  DoSatur=off
  Discrete-Time Integrator : DiscreteIntegrator  ExternalReset=either  SampleTime=-1  UpperSaturationLimit=0.3  LowerSaturationLimit=-0.3  ICPrevOutput=DiscIntNeverNeededParam  ICPrevScaledInput=DiscIntNeverNeededParam
  Gain : Gain
  Integral Gain : Gain  DisableCoverage=on  Gain=0
  Sum : Sum  Inputs=+++
  y : Outport  InitialOutput=0  VectorParamsAs1DForOutWhenUnconnected=off
  wires:
  reset_i/1 -> Discrete-Time Integrator/2
  Discrete-Time Integrator/1 -> Sum/2
  Discrete Derivative/1 -> Sum/3
  Sum/1 -> y/1
  Gain/1 -> Sum/1
  Derivative Gain/1 -> Discrete Derivative/1
  Integral Gain/1 -> Discrete-Time Integrator/1
  x/1 -> Derivative Gain/1, Integral Gain/1, Gain/1

== system SmallFixedWingUAVupperHIL/Controller/Subsystem4/PID_Altitude ==
  x : Inport
  reset_i : Inport  Port=2
  Derivative Gain : Gain  DisableCoverage=on  Gain=0  ParamMin=-100  ParamMax=100  OutMin=-100  OutMax=100
  Discrete Derivative : simulink/Discrete/Discrete Derivative  gainval=1.0  ICPrevScaledInput=0.0  OutMin=[]  OutMax=[]  OutDataType=fixdt(1, 16)  OutScaling=2^-10  DoSatur=off
  Discrete-Time Integrator : DiscreteIntegrator  ExternalReset=either  SampleTime=-1  ICPrevOutput=DiscIntNeverNeededParam  ICPrevScaledInput=DiscIntNeverNeededParam
  Gain : Gain  Gain=0.05
  Integral Gain : Gain  DisableCoverage=on  Gain=0
  Sum : Sum  Inputs=+++
  y : Outport  InitialOutput=0  VectorParamsAs1DForOutWhenUnconnected=off
  wires:
  x/1 -> Gain/1, Integral Gain/1, Derivative Gain/1
  Integral Gain/1 -> Discrete-Time Integrator/1
  Derivative Gain/1 -> Discrete Derivative/1
  Gain/1 -> Sum/1
  Sum/1 -> y/1
  Discrete Derivative/1 -> Sum/3
  Discrete-Time Integrator/1 -> Sum/2
  reset_i/1 -> Discrete-Time Integrator/2

== matlab function SmallFixedWingUAVupperHIL/Command/quat2eul ==
  data: q input; phi output; theta output; psi output
function [phi,theta,psi] = quat2eul(q)
% Conversion from Quaternion to Euler angles based on the PX4 Firmware
% v1.6.5 release.
% 
% Quaternion -> DCM -> Euler Angles
% INPUT:
%   q: Quaternion vector of the format: (a + bi + cj + dk)
% OUTPUT:
%   [phi,theta,psi]: Euler angles in radians.
% 
 
    a = q(1);
    b = q(2);
    c = q(3);
    d = q(4);

    aSq = a*a;
    bSq = b*b;
    cSq = c*c;
    dSq = d*d;

    d_pi2 = pi/2;

    % quaternion_to_dcm
    dcm00 = aSq + bSq - cSq - dSq;
    % dcm01 = 2*(b*c - a*d);
    dcm02 = 2*(a*c + b*d);
    dcm10 = 2*(b*c + a*d);
    % dcm11 = aSq - bSq + cSq - dSq;
    dcm12 = 2*(c*d - a*b);
    dcm20 = 2*(b*d - a*c);
    dcm21 = 2*(a*b + c*d);
    dcm22 = aSq - bSq - cSq + dSq;

    % dcm_to_euler
    theta = asin(-dcm20);
    if abs(theta - d_pi2) < 1.0e-3
        phi = single(0.0);
        psi = atan2(dcm12, dcm02);
    elseif abs(theta + d_pi2) < 1.0e-3
        phi = single(0.0);
        psi = atan2(-dcm12, -dcm02);
    else
        phi = atan2(dcm21, dcm22);
        psi = atan2(dcm10, dcm00);
    end

end

== matlab function SmallFixedWingUAVupperHIL/Controller/Information from Sensor/quat2eul ==
  data: q input; phi output; theta output; psi output
function [phi,theta,psi] = quat2eul(q)
% Conversion from Quaternion to Euler angles based on the PX4 Firmware
% v1.6.5 release.
% 
% Quaternion -> DCM -> Euler Angles
% INPUT:
%   q: Quaternion vector of the format: (a + bi + cj + dk)
% OUTPUT:
%   [phi,theta,psi]: Euler angles in radians.
% 
 
    a = q(1);
    b = q(2);
    c = q(3);
    d = q(4);

    aSq = a*a;
    bSq = b*b;
    cSq = c*c;
    dSq = d*d;

    d_pi2 = pi/2;

    % quaternion_to_dcm
    dcm00 = aSq + bSq - cSq - dSq;
    % dcm01 = 2*(b*c - a*d);
    dcm02 = 2*(a*c + b*d);
    dcm10 = 2*(b*c + a*d);
    % dcm11 = aSq - bSq + cSq - dSq;
    dcm12 = 2*(c*d - a*b);
    dcm20 = 2*(b*d - a*c);
    dcm21 = 2*(a*b + c*d);
    dcm22 = aSq - bSq - cSq + dSq;

    % dcm_to_euler
    theta = asin(-dcm20);
    if abs(theta - d_pi2) < 1.0e-3
        phi = single(0.0);
        psi = atan2(dcm12, dcm02);
    elseif abs(theta + d_pi2) < 1.0e-3
        phi = single(0.0);
        psi = atan2(-dcm12, -dcm02);
    else
        phi = atan2(dcm21, dcm22);
        psi = atan2(dcm10, dcm00);
    end

end

== matlab function SmallFixedWingUAVupperHIL/Command/MATLAB Function10 ==
  data: C input; vdv output
function vdv = track(C)
    vdv = [C(1),-C(2),0]';
end

== matlab function SmallFixedWingUAVupperHIL/Command/MATLAB Function11 ==
  data: C input; ada output
function ada = track(C)
    ada = [C(1),-C(2),0]';
end

== matlab function SmallFixedWingUAVupperHIL/Command/MATLAB Function12 ==
  data: n input; C output; t input; P input; U input
function C  = bspline_deboor(n,t,P,U)
%     validateattributes(n, {'numeric'}, {'positive','integer','scalar'});
    d = n;  % B-spline polynomial degree (1 for linear, 2 for quadratic, etc.)
%     validateattributes(t, {'numeric'}, {'real','vector'});
%     assert(all( t(2:end)-t(1:end-1) >= 0 ), 'bspline:deboor:InvalidArgumentValue', ...
%         'Knot vector values should be nondecreasing.');
%     validateattributes(P, {'numeric'}, {'real','2d'});
%     
%     if nargin < 4
%         U = linspace(t(d+1), t(end-d), 10*size(P,2));  % allocate points uniformly
%     elseif isscalar(U) && U > 1
%         validateattributes(U, {'numeric'}, {'positive','integer','scalar'});
%         U = linspace(t(d+1), t(end-d), U);  % allocate points uniformly
%     else
%         validateattributes(U, {'numeric'}, {'real','vector'});
%         assert(all( U >= t(d+1) & U <= t(end-d) ), 'bspline:deboor:InvalidArgumentValue', ...
%             'Value outside permitted knot vector value range.');
%     end
    
    m = size(P,1);  % dimension of control points
    t = t(:).';     % knot sequence
    U = U(:);
    S = sum(bsxfun(@eq, U, t), 2);  % multiplicity of u in t (0 <= s <= d+1)
    I = bspline_deboor_interval(U,t);
    if I>length(t)-d-1
       I=length(t)-d-1;
    end
    if I == -1
        I = length(t)-d-1;
    end
    Pk = zeros(m,d+40,d+40);
    a = zeros(d+40,d+40);
    
    C = zeros(size(P,1), numel(U));
    for j = 1 : numel(U)
        u = U(j);
        s = S(j);
        ix = I(j);
        Pk(:) = 0;
        a(:) = 0;
    
        % identify d+1 relevant control points
%         Pk(:, (ix-d):(ix-s), 1) = P(:, (ix-d):(ix-s));
        h = d - s;
        if h > 0 
            Pk(:, (ix-d):(ix-s), 1) = P(:, (ix-d):(ix-s));
        end
        if h > 0
            % de Boor recursion formula
            for r = 1 : h
                q = ix-1;
                for i = (q-d+r) : (q-s)
                    a(i+1,r+1) = (u-t(i+1)) / (t(i+d-r+1+1)-t(i+1));
                    Pk(:,i+1,r+1) = (1-a(i+1,r+1)) * Pk(:,i,r) + a(i+1,r+1) * Pk(:,i+1,r);
                end
            end
            C(:,j) = Pk(:,ix-s,d-s+1);  % extract value from triangular computation scheme
        elseif ix == numel(t)  % last control point is a special case
            C(:,j) = P(:,end);
        else
            C(:,j) = P(:,ix-d);
        end
    end
end

function ix = bspline_deboor_interval(u,t)
% Index of knot in knot sequence not less than the value of u.
% If knot has multiplicity greater than 1, the highest index is returned.
    for i = 1:length(t)
        if t(i)>u
            ix = i;
            return
        end
    end
    ix = -1;
end
% function ix = bspline_deboor_interval(u,t)
% % Index of knot in knot sequence not less than the value of u.
% % If knot has multiplicity greater than 1, the highest index is returned.
% 
% i = bsxfun(@ge, u, t) & bsxfun(@lt, u, [t(2:end) 2*t(end)]);  % indicator of knot interval in which u is
% [row,col] = find(i);
% [row,ind] = sort(row);  % restore original order of data points
% ix = col(ind);
% end

== matlab function SmallFixedWingUAVupperHIL/Command/MATLAB Function13 ==
  data: p output; order input; dknots output; knots input; ctrl input; dctrl output
function [p, dknots, dctrl] = bspline_deriv(order, knots, ctrl)
    p = order;
    tmp = size(ctrl);
    n = tmp(2)-1;
    dim = tmp(1);
    
    % derivative knots
    dknots = knots(2:max(size(knots))-1);
    
    % derivative control points
    dctrl = zeros(dim,n);
    for i = 1 : n
        dctrl(:,i) = (p / (knots(i+p+1) - knots(i+1))) * (ctrl(:,i+1) - ctrl(:,i));
    end
    p = order-1;
end

== matlab function SmallFixedWingUAVupperHIL/Command/MATLAB Function14 ==
  data: p output; order input; dknots output; knots input; ctrl input; dctrl output
function [p, dknots, dctrl] = bspline_deriv(order, knots, ctrl)
    p = order;
    tmp = size(ctrl);
    n = tmp(2)-1;
    dim = tmp(1);
    
    % derivative knots
    dknots = knots(2:max(size(knots))-1);
    
    % derivative control points
    dctrl = zeros(dim,n);
    for i = 1 : n
        dctrl(:,i) = (p / (knots(i+p+1) - knots(i+1))) * (ctrl(:,i+1) - ctrl(:,i));
    end
    p = order-1;
end

== matlab function SmallFixedWingUAVupperHIL/Command/MATLAB Function15 ==
  data: C input; xdx output
function xdx = track(C)
    xdx = [C(1),-C(2),0]';
end

== matlab function SmallFixedWingUAVupperHIL/Command/MATLAB Function7 ==
  data: n input; C output; t input; P input; U input
function C = bspline_deboor(n,t,P,U)
%     validateattributes(n, {'numeric'}, {'positive','integer','scalar'});
    d = n;  % B-spline polynomial degree (1 for linear, 2 for quadratic, etc.)
%     validateattributes(t, {'numeric'}, {'real','vector'});
%     assert(all( t(2:end)-t(1:end-1) >= 0 ), 'bspline:deboor:InvalidArgumentValue', ...
%         'Knot vector values should be nondecreasing.');
%     validateattributes(P, {'numeric'}, {'real','2d'});
%     
%     if nargin < 4
%         U = linspace(t(d+1), t(end-d), 10*size(P,2));  % allocate points uniformly
%     elseif isscalar(U) && U > 1
%         validateattributes(U, {'numeric'}, {'positive','integer','scalar'});
%         U = linspace(t(d+1), t(end-d), U);  % allocate points uniformly
%     else
%         validateattributes(U, {'numeric'}, {'real','vector'});
%         assert(all( U >= t(d+1) & U <= t(end-d) ), 'bspline:deboor:InvalidArgumentValue', ...
%             'Value outside permitted knot vector value range.');
%     end
    
    m = size(P,1);  % dimension of control points
    t = t(:).';     % knot sequence
    U = U(:);
    S = sum(bsxfun(@eq, U, t), 2);  % multiplicity of u in t (0 <= s <= d+1)
    I = bspline_deboor_interval(U,t);
    if I>length(t)-d-1
       I=length(t)-d-1;
    end
    if I == -1
        I = length(t)-d-1;
    end
    Pk = zeros(m,d+40,d+40);
    a = zeros(d+40,d+40);
    
    C = zeros(size(P,1), numel(U));
    for j = 1 : numel(U)
        u = U(j);
        s = S(j);
        ix = I(j);
        Pk(:) = 0;
        a(:) = 0;
    
        % identify d+1 relevant control points
%         Pk(:, (ix-d):(ix-s), 1) = P(:, (ix-d):(ix-s));
        h = d - s;
        if h > 0 
            Pk(:, (ix-d):(ix-s), 1) = P(:, (ix-d):(ix-s));
        end
        if h > 0
            % de Boor recursion formula
            for r = 1 : h
                q = ix-1;
                for i = (q-d+r) : (q-s)
                    a(i+1,r+1) = (u-t(i+1)) / (t(i+d-r+1+1)-t(i+1));
                    Pk(:,i+1,r+1) = (1-a(i+1,r+1)) * Pk(:,i,r) + a(i+1,r+1) * Pk(:,i+1,r);
                end
            end
            C(:,j) = Pk(:,ix-s,d-s+1);  % extract value from triangular computation scheme
        elseif ix == numel(t)  % last control point is a special case
            C(:,j) = P(:,end);
        else
            C(:,j) = P(:,ix-d);
        end
    end
end

function ix = bspline_deboor_interval(u,t)
% Index of knot in knot sequence not less than the value of u.
% If knot has multiplicity greater than 1, the highest index is returned.
    for i = 1:length(t)
        if t(i)>u
            ix = i;
            return
        end
    end
    ix = -1;
end

% function ix = bspline_deboor_interval(u,t)
% % Index of knot in knot sequence not less than the value of u.
% % If knot has multiplicity greater than 1, the highest index is returned.
% 
% i = bsxfun(@ge, u, t) & bsxfun(@lt, u, [t(2:end) 2*t(end)]);  % indicator of knot interval in which u is
% [row,col] = find(i);
% [row,ind] = sort(row);  % restore original order of data points
% ix = col(ind);
% end
